simulink model "Current_AD"  (R2022b)
settings: Solver=FixedStepAuto  StartTime=0.0  StopTime=10.0  FixedStep=Ts_Sensor  RelTol=1e-3
undefined symbols (not defined in the file): ADCBit, Current_Gain, Current_Offset, Ts_Sensor, Vcc
settings Model: Creator=BEDNASA  LastModifiedBy=HENRIE2
settings SolverCC: AlgebraicLoopSolver=TrustRegion
settings DebuggingCC: UnconnectedInputMsg=warning  UnconnectedOutputMsg=warning  UnconnectedLineMsg=warning  SFMachineParentedDataDiag=warning
settings ModelReferenceCC: EnableRefExpFcnMdlSchedulingChecks=on

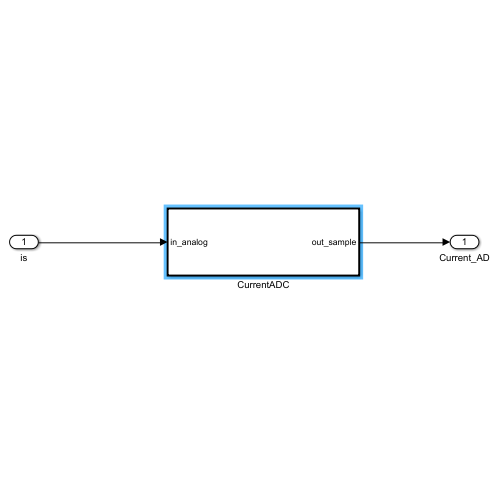
[thumbnail: Simulink's stored preview of the top-level diagram]
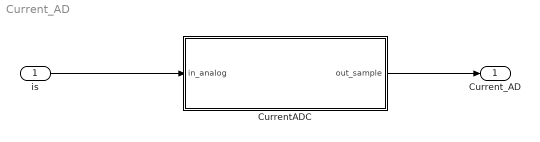
== system Current_AD ==
  is : Inport
  CurrentADC : Subsystem  TreatAsAtomicUnit=on  SystemSampleTime=Ts_Sensor
  Current_AD : Outport
  wires:
  CurrentADC/1(out_sample) -> Current_AD/1
  is/1 -> CurrentADC/1(in_analog)

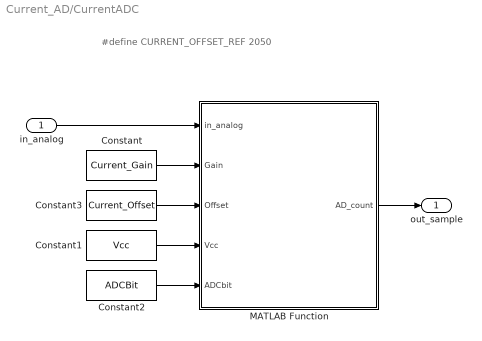
== system Current_AD/CurrentADC ==
  note: #define CURRENT_OFFSET_REF 2050
  in_analog : Inport
  Constant : Constant  Value=Current_Gain
  Constant1 : Constant  Value=Vcc
  Constant2 : Constant  Value=ADCBit
  Constant3 : Constant  Value=Current_Offset
  MATLAB Function : MATLAB Function  TreatAsAtomicUnit=on
  out_sample : Outport
  wires:
  in_analog/1 -> MATLAB Function/1(in_analog)
  MATLAB Function/1(AD_count) -> out_sample/1
  Constant/1 -> MATLAB Function/2(Gain)
  Constant3/1 -> MATLAB Function/3(Offset)
  Constant1/1 -> MATLAB Function/4(Vcc)
  Constant2/1 -> MATLAB Function/5(ADCbit)

== matlab function Current_AD/CurrentADC/MATLAB Function ==
  data: in_analog input; AD_count output; Gain input; Offset input; Vcc input; ADCbit input
function AD_count  = GetADCRawData(in_analog, Gain, Offset, Vcc, ADCbit)
%% Sensor model with ADC
% Sensor voltage equation V_out = Gain * in_analog + Offset

V_out = Gain * in_analog + Offset;

if (V_out > Vcc)
    V_out = Vcc;
elseif (V_out < 0)
    V_out = 0;
end

%% AD Counts
AD_count = round((V_out/Vcc) * (2^ADCbit));
end
